simulink model "Razomkn"  (R2023a)
settings: Solver=VariableStepAuto  StartTime=0.0  StopTime=10.0  RelTol=1e-3
settings Model: Creator=ycheb  LastModifiedBy=ycheb

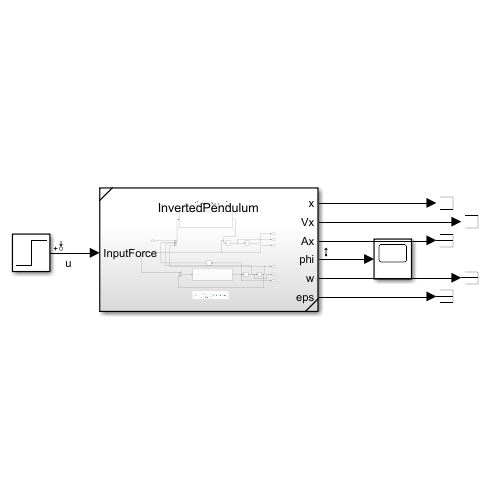
[thumbnail: Simulink's stored preview of the top-level diagram]
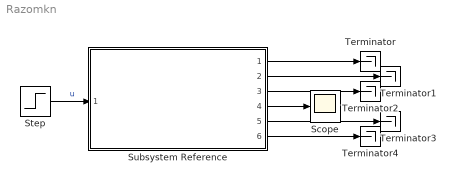
== system Razomkn ==
  Scope : Scope
  Step : Step  SampleTime=0
  Subsystem Reference : Subsystem  ReferencedSubsystem=InvertedPendulum
  Terminator{,1..4} (5 alike) : Terminator
  wires:
  Step/1 -> Subsystem Reference/1  "u"
  Subsystem Reference/4 -> Scope/1
  Subsystem Reference/2 -> Terminator1/1
  Subsystem Reference/1 -> Terminator/1
  Subsystem Reference/3 -> Terminator2/1
  Subsystem Reference/5 -> Terminator3/1
  Subsystem Reference/6 -> Terminator4/1
